simulink model "PVHome"  (R2022b)
settings: Solver=FixedStepDiscrete  StartTime=0.0  StopTime=2  FixedStep=5e-6  RelTol=1e-3
undefined symbols (not defined in the file): Ion, Lithium
libraries: spsSeriesRLCBranchLib x175, spsBreakerLib x103, spsPWMGeneratorDCDCLib x94, spsThyristorLib x78, slpidlib x72, spsIGBTDiodeLib x62, spsThreePhaseVIMeasurementLib x59, spsThreePhaseBreakerLib x45, spsVoltageMeasurementLib x45, spsDiodeLib x39, spsThreePhaseParallelRLCBranchLib x38, spsMosfetLib x32
(part 6 of 16)

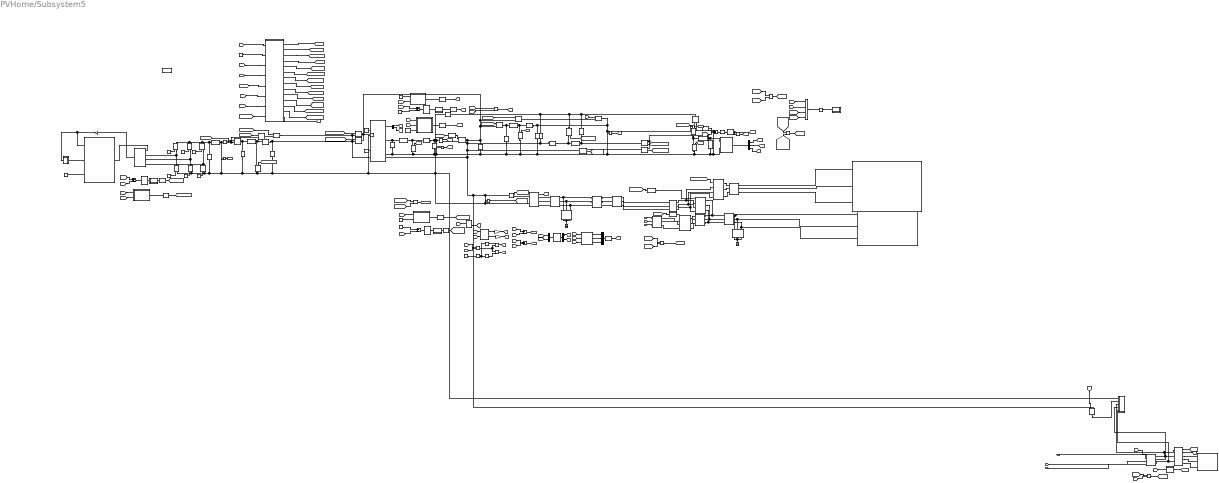
== system PVHome/Subsystem5 ==
  note: CONSUMER
  note: LOAD HOUSE
  note: TRADER GRID
  note: consider a such a language so as to make the system to understand
      |
      | hence consider a system with values range (around keep it as heat) as 0 to 1 but it has to show until 200 degrees.
      |
      | so we divide 1/200 and get 0.005
      |
      | each dividision becomes 0.005
      | 1 is 0.005
      | 2 is 0.01
      | 3 is 0.015
      | 4 is 0.02
      |
      |
      | like that
      | 0.5 becomes 100
      |
      | why not till 200?
      |
      |
      | maybe can increase cost, space like that.
      | hence we program it.
      |
      | consider an integral controller, the default set needed input is around 120 degree and in 0 to 1 scale of 200 divisions (max 200 degree means and 1 is 200).
      |
      | we only get 70 and its 0.35 in set range
      |
      | but we need 120 ie 0.6
      |
      | so the difference becomes error E(t)=50
      | (1/200) integral of E(t) at 0 to t at t=1, it becomes 50(1)/200= 0.25.
      |
      | hence 0.25 must be added to the 0.35 to make it 0.6. so the 0.25 is slowly added to the system with 0.35 and makes it 0.6.
      |
      | after it becomes 0.6, the output is 120 and error is 0 and 0.6 is neither lessened or addened due to past system memory.
      |
      |
      | therefore the 0 to 1 with 200 divisions is a kind of thing that set to make the system understand the human mind from outside.
      |
      | again why not 0 to 200?, human designes the system, consider it has been designed like this.
  note: for how much seconds the output is produced is solver
      | if for 5e-3 seconds in solver a output is loaded for each of 5e-3 seconds
      |
      |
      | powergui is needed because the power system blocks could not be solved using the normal solver.
      |
      | we need a seperate ones like power gui to regulate output within given times.
      |
      | those both normla global solver and the gui must sink such as to make the functions and output possible.
      |
      | or the system cant produce output
      |
      | the gui suppose runs at 4e-3 and normal at 5e-3
      |
      | the output at power system is produced once 4e-3 s
      | and that output is loaded in 5e-3 seconds
      |
      |
      | the synchronzation problem occurs
  note: REAL GRID
  note: Negative meetup
  note: positive total
  note: less act
  note: when th produced voltage supply becomes less than the thought of battery voltage
  note: when the produced voltage becomes high comparitive to the battery
  note: 60
  note: 150
  note: 45
  note: 60
  note: 15
  note: Buck conv
  note: Boost conv
  note: WIND TURBINES
  note: Dc to ac asnd also the Power factor scrutnification
  note: This is for random speeds
  note: Look, the Pu values are nothing but the like example the if at all value is 1, means the value of 3.3 KW is divided into 10 parts. if at all the 0.1 means 10% of 3.3Kw.
      | In turn in the base wind the maximum is 12 and the PU is 1.3, the 13 is divided into 13 parts.
  note: Basically this capacitor works in a way like if at all there is the igbt closed, the capacior will make the higher potential say 190 V and the anode of diode will be 0 V and this makes the capacitor higher potential and anode lower potential and hence reverse bias. After that, when the power flows inside (anode) it, the becomes 230 V suppose, this will surely be higher potential and the 190V will be lower potental and the power flows in forward bias
  note: the tan of the phi and the pi power is Q
  note: Basically in pi controller consider the Default or setted ones are like 120 degree celcius. If at all the feedback input is around 70 degree celcius, the error becomes like 50 degrees. this will go in and the feedback input's magnitude will be considered as the ki as 1/70 and the integral will be from 0 to t as limits and the {E(t)=50}dt inside. Then the 0.42 of error produces and this will make the system increase the 0.42 percet or something. (considering 0.7 before) and goes to 1.142. This will make system at120 degree celcius. This inturn returns as feedback input and the error is 0 and the 1.142 doesnet decrease or increase due to system memory.
  note: basically pitch angle is the one which. Before that, the windmill soins in certain way and in turn the wings of the windmill also rotates. basically like earth rotation is wings and the earth's revolution is the spinning of wings.
      |
      | The pitch angle must be 0 for maximum speed and 90 for minimum speed.
      | the pitch controller is deisgned in such a way that itg included the Pi control mechanism inside it.
      | When the error comes in the PI, kt converts suitable values and proceeeds with into the system via out.
      | After that if at all the output of the system and the refrecnce makes the error 0, thr picth degree stays at specific increases point. or decresaed point.
      |
      |
      |
      | If consider taht the error is  neagtive, then the speed is more than default or setted speed. this makes the RPM to spin fast more than rated speed and making it to damage. Even though the power will wont be produced more , but causes physical damage. Hence that negative causes to increase the pitch angle to certain level (basicallyturn) and make it spin less.
  note: think like a right angled triangle. the hypotenuse as apprarent power, the vertical ones as the VI cos phi that is active power, and the sine ones VI sin phi as the reactive power,
  note: if you remove the cos phi, you will just get the apprarent power which is combination of the active power and reactive power
  note: Trading grid
  note: House Load DC to AC conversion
  note: Battery recharge and discharge system
  note: PV Array System
  note: Centralized system
  note: HOUSE LOAD
  note: so basically these are used like for solving equations. Each type of equation has a each need. the power electronics and other stuff has some other discrete mode and need ans other stuff.
      | the thing at bottom right will evaluate some signal equation only not deep power electronics and stuff.
      | to match those we keep that power gui block. continious signals will help in bothcases and will evaluate.
      | the time is which 5e-6 like how much time interval thse will work
      | the each equation is getting evaluated in this much small interval.
      | the pwm signal around goes upto 50000 cycles in real human second according to this solver
  note: this and the power gui matches then the power system specialized will be resolvered in this sepcific timem like 5e-6
  note: the solver time like 5e-6 will solve each and next equations in this specific time
  note: Like without the power gui the simulink cant simulate the power specializized systems
  note: so these power gui blocks and the solvers are used in such a away that the functions are done
  note: because power (current flows from higher potential to lower potentail
  note: here in capacitor, when the other part of diode is higher potential and this capacior has lower potential, the power flows, if its vice versa, the capacitor side becomes the higher potential and the other side becomes lower potential
  note: breaker analogy
  note: 1 open
  note: 0 closed
  note: Q=VItan phi
  note: phi is cos inverse
  note: Power factor = cos phi
  note: this must activate when there is pv power availablity
  note: this must activate when no power is available in the pv or no sufficient power available in PV
  Add : Sum  Inputs=+-
  Add2 : Sum  Inputs=+-
  Add3 : Sum  Inputs=+-
  Battery : spsBatteryLib/Battery  BatType=Lithium-Ion  ShowTempParam=off  ThermalPreset=no  ShowAgeParam=off  NomV=60  NomQ=50  SOC=50  Batt_Tr=1  PresetModel=off  MaxQ=50  MinV=45  FullV=69.8392  Dis_rate=21.7391  R=0.012  Normal_OP=45.2174  expZone="[64.8232      2.45652]"  current=[6.5 13 32.5]  Units=Time  Tci=20  NomT=20  T2=-30  MaxQ2=4.8  FullV2=7.1  Normal_OP2=5.655  expZone2="[6.58           1]"  Rca=0.6  ti=2000  Dp=0  Neq0=0  Tsim=1e6  Ta1=25  Qeol=5.4*0.9  Reol=0.013333*1.2  Char_age=[2.3478, 3]  Dis_age=[2.3478, 10]  N1=1500  N2=10500  N3=1000  N4=1400  Ta2=45  N5=950
  Breaker{1..10,19} (11 alike) : spsBreakerLib/Breaker  InitialState=0  SwitchingTimes="[1/60  5/60]"  External=on  BreakerResistance=0.01  SnubberResistance=1e6  SnubberCapacitance=inf  Measurements=None  MoreParameters=on  NoBreakLoop=off
  Bus Creator : BusCreator  Inputs=3
  Bus Selector : BusSelector  OutputSignals=V_PV,I_PV
  Bus Selector1 : BusSelector  OutputSignals=SOC (%),Current (A),Voltage (V)
  CAPACITOR {1,7,9..10,14} (5 alike) : spsSeriesRLCBranchLib/Series RLC Branch  LConnTagsString=__new0  RConnTagsString=__new0  BranchType=RC  Resistance=1e-4  Inductance=5e-3  SetiL0=off  InitialCurrent=0  Capacitance=2000e-3  Setx0=off  InitialVoltage=0  Measurements=None
  CAPACITOR {2,8,11,13,18} (5 alike) : spsSeriesRLCBranchLib/Series RLC Branch  LConnTagsString=__new0  RConnTagsString=__new0  BranchType=RL  Resistance=1e-4  Inductance=1e-3  SetiL0=off  InitialCurrent=0  Capacitance=100e-6  Setx0=off  InitialVoltage=0  Measurements=None
  CAPACITOR {3..5,12,16..17,19} (7 alike) : spsSeriesRLCBranchLib/Series RLC Branch  LConnTagsString=__new0  RConnTagsString=__new0  BranchType=RC  Resistance=1e-4  Inductance=5e-3  SetiL0=off  InitialCurrent=0  Capacitance=100e-6  Setx0=off  InitialVoltage=0  Measurements=None
  CAPACITOR 6 : spsSeriesRLCBranchLib/Series RLC Branch  LConnTagsString=__new0  RConnTagsString=__new0  BranchType=RL  Resistance=1e-4  Inductance=13e-3  SetiL0=off  InitialCurrent=0  Capacitance=100e-6  Setx0=off  InitialVoltage=0  Measurements=None
  Centralized System : MATLAB Function  TreatAsAtomicUnit=on
  Constant : Constant  Value=1000
  Constant1 : Constant  Value=25
  Constant2 : Constant  Value=0.005
  Constant3 : Constant  Value=60
  Constant4 : Constant  Value=2300
  Constant5 : Constant  Value=25
  Constant6 : Constant  Value=60
  Current Measurement1 : spsCurrentMeasurementLib/Current Measurement  PhasorSimulation=off  OutputType=Complex  PSBequivalent=0
  Current Measurement2 : spsCurrentMeasurementLib/Current Measurement  PhasorSimulation=off  OutputType=Complex  PSBequivalent=0
  Current Measurement3 : spsCurrentMeasurementLib/Current Measurement  PhasorSimulation=off  OutputType=Complex  PSBequivalent=0
  Data Type Conversion : DataTypeConversion  OutDataTypeStr=boolean  SaturateOnIntegerOverflow=off  RndMeth=Floor
  Data Type Conversion1 : DataTypeConversion  OutDataTypeStr=boolean  SaturateOnIntegerOverflow=off  RndMeth=Floor
  Data Type Conversion2 : DataTypeConversion  OutDataTypeStr=boolean  SaturateOnIntegerOverflow=off  RndMeth=Floor
  Demux : Demux  Outputs=2
  Diode{1..4} (4 alike) : spsDiodeLib/Diode  Ron=0.001  Lon=0  Vf=0.8  IC=0  UseSnubber=0  Rs=500  Cs=250e-9  Measurements=off
  Discrete PID Controller : slpidlib/PID Controller  Controller=PI  Form=Parallel  TimeDomain=Discrete-time  UseExternalTs=off  SampleTime=1e-5  IntegratorMethod=Forward Euler  FilterMethod=Forward Euler  ControllerParametersSource=internal  P=0.01  I=1  UseKiTs=off  D=0  N=100  UseFilter=on  TunerSelectOption=Transfer Function Based (PID Tuner App)  InitialConditionSource=internal  InitialConditionForIntegrator=0  InitialConditionForFilter=0  DifferentiatorICPrevScaledInput=0  ExternalReset=none  TrackingMode=off  Kt=1  LimitOutput=on  SatLimitsSource=internal  UpperSaturationLimit=1.1  LowerSaturationLimit=-1.1  LinearizeAsGain=off  AntiWindupMode=none  Kb=1  LimitIntegrator=off  UpperIntegratorSaturationLimit=inf  LowerIntegratorSaturationLimit=-inf  POutMin=[]  POutMax=[]  IOutMin=[]  IOutMax=[]  DOutMin=[]  DOutMax=[]  NOutMin=[]  NOutMax=[]  SumOutMin=[]  SumOutMax=[]  SaturationOutMin=[]  SaturationOutMax=[]  PParamMin=[]  PParamMax=[]  IParamMin=[]  IParamMax=[]  DParamMin=[]  DParamMax=[]  NParamMin=[]  NParamMax=[]  KbParamMin=[]  KbParamMax=[]  KtParamMin=[]  KtParamMax=[]  KbOutMin=[]  KbOutMax=[]  KtOutMin=[]  KtOutMax=[]  IntegratorOutMin=[]  IntegratorOutMax=[]  FilterOutMin=[]  FilterOutMax=[]  SumI1OutMin=[]  SumI1OutMax=[]  SumI2OutMin=[]  SumI2OutMax=[]  SumI3OutMin=[]  SumI3OutMax=[]  SumI4OutMin=[]  SumI4OutMax=[]  SumDOutMin=[]  SumDOutMax=[]  DifferentiatorOutMin=[]  DifferentiatorOutMax=[]  FilterDiffOutCoefMin=[]  FilterDiffOutCoefMax=[]  ReciprocalOutMin=[]  ReciprocalOutMax=[]  SumDenOutMin=[]  SumDenOutMax=[]  SumNumOutMin=[]  SumNumOutMax=[]  DivideOutMin=[]  DivideOutMax=[]  UdiffTsProdOutMin=[]  UdiffTsProdOutMax=[]  NTsProdOutMin=[]  NTsProdOutMax=[]  UintegralTsProdOutMin=[]  UintegralTsProdOutMax=[]  UngainTsProdOutMin=[]  UngainTsProdOutMax=[]  ClampingZeroOutDataTypeStr=Inherit: Inherit via back propagation  ClampingZeroOutMin=[]  ClampingZeroOutMax=[]  FilterDenConstantOutDataTypeStr=Inherit: Inherit via back propagation  FilterDenConstantOutMin=[]  FilterDenConstantOutMax=[]  PCopyOutDataTypeStr=Inherit: Inherit via back propagation  PCopyOutMin=[]  PCopyOutMax=[]  NCopyOutDataTypeStr=Inherit: Inherit via back propagation  NCopyOutMin=[]  NCopyOutMax=[]  IntegratorContinuousStateAttributes=''  IntegratorStateMustResolveToSignalObject=off  IntegratorRTWStateStorageClass=Auto  FilterContinuousStateAttributes=''  FilterStateMustResolveToSignalObject=off  FilterRTWStateStorageClass=Auto  ParallelPVariant=InternalParameters  IdealPVariant=Disabled  IVariant=InternalParameters  DVariant=Disabled  IntegratorVariant=Discrete  SatVariant=Enabled  AWVariant=Passthrough  PCopyVariant=Disabled  TRVariant=Disabled  FdbkBlocksVariant=Forward  IdealPFdbkVariant=Disabled  SatFdbkVariant=Disabled  DerivativeFilterVariant=Disabled  NVariant=Disabled  NCopyVariant=Disabled_SignalSpec  FilterICVariant=Disabled  IntegratorICVariant=InternalICs  ExternalResetVariant=Disabled  TRSumVariant=Passthrough  SumFdbkVariant=Disabled  SumVariant=Sum_PI  TsampFilterVariant=InternalTs  TsampNgainVariant=Passthrough  TsampIntegralVariant=Passthrough  ExternalSaturationOutDataTypeStr=Inherit: Same as second input
      settings: LibrarySourceBlock=simulink/Discrete/Discrete PID Controller
  Discrete PID Controller1 : slpidlib/PID Controller  Controller=PI  Form=Parallel  TimeDomain=Discrete-time  UseExternalTs=off  SampleTime=-1  IntegratorMethod=Forward Euler  FilterMethod=Forward Euler  ControllerParametersSource=internal  P=1  I=1  UseKiTs=off  D=0  N=100  UseFilter=on  TunerSelectOption=Transfer Function Based (PID Tuner App)  InitialConditionSource=internal  InitialConditionForIntegrator=0  InitialConditionForFilter=0  DifferentiatorICPrevScaledInput=0  ExternalReset=none  TrackingMode=off  Kt=1  LimitOutput=off  SatLimitsSource=internal  UpperSaturationLimit=inf  LowerSaturationLimit=-inf  LinearizeAsGain=off  AntiWindupMode=none  Kb=1  LimitIntegrator=off  UpperIntegratorSaturationLimit=inf  LowerIntegratorSaturationLimit=-inf  POutMin=[]  POutMax=[]  IOutMin=[]  IOutMax=[]  DOutMin=[]  DOutMax=[]  NOutMin=[]  NOutMax=[]  SumOutMin=[]  SumOutMax=[]  SaturationOutMin=[]  SaturationOutMax=[]  PParamMin=[]  PParamMax=[]  IParamMin=[]  IParamMax=[]  DParamMin=[]  DParamMax=[]  NParamMin=[]  NParamMax=[]  KbParamMin=[]  KbParamMax=[]  KtParamMin=[]  KtParamMax=[]  KbOutMin=[]  KbOutMax=[]  KtOutMin=[]  KtOutMax=[]  IntegratorOutMin=[]  IntegratorOutMax=[]  FilterOutMin=[]  FilterOutMax=[]  SumI1OutMin=[]  SumI1OutMax=[]  SumI2OutMin=[]  SumI2OutMax=[]  SumI3OutMin=[]  SumI3OutMax=[]  SumI4OutMin=[]  SumI4OutMax=[]  SumDOutMin=[]  SumDOutMax=[]  DifferentiatorOutMin=[]  DifferentiatorOutMax=[]  FilterDiffOutCoefMin=[]  FilterDiffOutCoefMax=[]  ReciprocalOutMin=[]  ReciprocalOutMax=[]  SumDenOutMin=[]  SumDenOutMax=[]  SumNumOutMin=[]  SumNumOutMax=[]  DivideOutMin=[]  DivideOutMax=[]  UdiffTsProdOutMin=[]  UdiffTsProdOutMax=[]  NTsProdOutMin=[]  NTsProdOutMax=[]  UintegralTsProdOutMin=[]  UintegralTsProdOutMax=[]  UngainTsProdOutMin=[]  UngainTsProdOutMax=[]  ClampingZeroOutDataTypeStr=Inherit: Inherit via back propagation  ClampingZeroOutMin=[]  ClampingZeroOutMax=[]  FilterDenConstantOutDataTypeStr=Inherit: Inherit via back propagation  FilterDenConstantOutMin=[]  FilterDenConstantOutMax=[]  PCopyOutDataTypeStr=Inherit: Inherit via back propagation  PCopyOutMin=[]  PCopyOutMax=[]  NCopyOutDataTypeStr=Inherit: Inherit via back propagation  NCopyOutMin=[]  NCopyOutMax=[]  IntegratorContinuousStateAttributes=''  IntegratorStateMustResolveToSignalObject=off  IntegratorRTWStateStorageClass=Auto  FilterContinuousStateAttributes=''  FilterStateMustResolveToSignalObject=off  FilterRTWStateStorageClass=Auto  ParallelPVariant=InternalParameters  IdealPVariant=Disabled  IVariant=InternalParameters  DVariant=Disabled  IntegratorVariant=Discrete  SatVariant=Disabled  AWVariant=Passthrough  PCopyVariant=Disabled  TRVariant=Disabled  FdbkBlocksVariant=Forward  IdealPFdbkVariant=Disabled  SatFdbkVariant=Disabled  DerivativeFilterVariant=Disabled  NVariant=Disabled  NCopyVariant=Disabled_SignalSpec  FilterICVariant=Disabled  IntegratorICVariant=InternalICs  ExternalResetVariant=Disabled  TRSumVariant=Passthrough  SumFdbkVariant=Disabled  SumVariant=Sum_PI  TsampFilterVariant=InternalTs  TsampNgainVariant=Passthrough  TsampIntegralVariant=Passthrough  ExternalSaturationOutDataTypeStr=Inherit: Same as second input
      settings: LibrarySourceBlock=simulink/Discrete/Discrete PID Controller
  Discrete PID Controller3 : slpidlib/PID Controller  Controller=PI  Form=Parallel  TimeDomain=Discrete-time  UseExternalTs=off  SampleTime=1e-5  IntegratorMethod=Forward Euler  FilterMethod=Forward Euler  ControllerParametersSource=internal  P=0  I=0.01667  UseKiTs=off  D=0  N=100  UseFilter=on  TunerSelectOption=Transfer Function Based (PID Tuner App)  InitialConditionSource=internal  InitialConditionForIntegrator=0  InitialConditionForFilter=0  DifferentiatorICPrevScaledInput=0  ExternalReset=none  TrackingMode=off  Kt=1  LimitOutput=on  SatLimitsSource=internal  UpperSaturationLimit=1.1  LowerSaturationLimit=-1.1  LinearizeAsGain=off  AntiWindupMode=none  Kb=1  LimitIntegrator=off  UpperIntegratorSaturationLimit=inf  LowerIntegratorSaturationLimit=-inf  POutMin=[]  POutMax=[]  IOutMin=[]  IOutMax=[]  DOutMin=[]  DOutMax=[]  NOutMin=[]  NOutMax=[]  SumOutMin=[]  SumOutMax=[]  SaturationOutMin=[]  SaturationOutMax=[]  PParamMin=[]  PParamMax=[]  IParamMin=[]  IParamMax=[]  DParamMin=[]  DParamMax=[]  NParamMin=[]  NParamMax=[]  KbParamMin=[]  KbParamMax=[]  KtParamMin=[]  KtParamMax=[]  KbOutMin=[]  KbOutMax=[]  KtOutMin=[]  KtOutMax=[]  IntegratorOutMin=[]  IntegratorOutMax=[]  FilterOutMin=[]  FilterOutMax=[]  SumI1OutMin=[]  SumI1OutMax=[]  SumI2OutMin=[]  SumI2OutMax=[]  SumI3OutMin=[]  SumI3OutMax=[]  SumI4OutMin=[]  SumI4OutMax=[]  SumDOutMin=[]  SumDOutMax=[]  DifferentiatorOutMin=[]  DifferentiatorOutMax=[]  FilterDiffOutCoefMin=[]  FilterDiffOutCoefMax=[]  ReciprocalOutMin=[]  ReciprocalOutMax=[]  SumDenOutMin=[]  SumDenOutMax=[]  SumNumOutMin=[]  SumNumOutMax=[]  DivideOutMin=[]  DivideOutMax=[]  UdiffTsProdOutMin=[]  UdiffTsProdOutMax=[]  NTsProdOutMin=[]  NTsProdOutMax=[]  UintegralTsProdOutMin=[]  UintegralTsProdOutMax=[]  UngainTsProdOutMin=[]  UngainTsProdOutMax=[]  ClampingZeroOutDataTypeStr=Inherit: Inherit via back propagation  ClampingZeroOutMin=[]  ClampingZeroOutMax=[]  FilterDenConstantOutDataTypeStr=Inherit: Inherit via back propagation  FilterDenConstantOutMin=[]  FilterDenConstantOutMax=[]  PCopyOutDataTypeStr=Inherit: Inherit via back propagation  PCopyOutMin=[]  PCopyOutMax=[]  NCopyOutDataTypeStr=Inherit: Inherit via back propagation  NCopyOutMin=[]  NCopyOutMax=[]  IntegratorContinuousStateAttributes=''  IntegratorStateMustResolveToSignalObject=off  IntegratorRTWStateStorageClass=Auto  FilterContinuousStateAttributes=''  FilterStateMustResolveToSignalObject=off  FilterRTWStateStorageClass=Auto  ParallelPVariant=InternalParameters  IdealPVariant=Disabled  IVariant=InternalParameters  DVariant=Disabled  IntegratorVariant=Discrete  SatVariant=Enabled  AWVariant=Passthrough  PCopyVariant=Disabled  TRVariant=Disabled  FdbkBlocksVariant=Forward  IdealPFdbkVariant=Disabled  SatFdbkVariant=Disabled  DerivativeFilterVariant=Disabled  NVariant=Disabled  NCopyVariant=Disabled_SignalSpec  FilterICVariant=Disabled  IntegratorICVariant=InternalICs  ExternalResetVariant=Disabled  TRSumVariant=Passthrough  SumFdbkVariant=Disabled  SumVariant=Sum_PI  TsampFilterVariant=InternalTs  TsampNgainVariant=Passthrough  TsampIntegralVariant=Passthrough  ExternalSaturationOutDataTypeStr=Inherit: Same as second input
      settings: LibrarySourceBlock=simulink/Discrete/Discrete PID Controller
  Discrete PID Controller4 : slpidlib/PID Controller  Controller=PI  Form=Parallel  TimeDomain=Discrete-time  UseExternalTs=off  SampleTime=1e-5  IntegratorMethod=Forward Euler  FilterMethod=Forward Euler  ControllerParametersSource=internal  P=0  I=0.01  UseKiTs=off  D=0  N=100  UseFilter=on  TunerSelectOption=Transfer Function Based (PID Tuner App)  InitialConditionSource=internal  InitialConditionForIntegrator=0  InitialConditionForFilter=0  DifferentiatorICPrevScaledInput=0  ExternalReset=none  TrackingMode=off  Kt=1  LimitOutput=on  SatLimitsSource=internal  UpperSaturationLimit=1.1  LowerSaturationLimit=-1.1  LinearizeAsGain=off  AntiWindupMode=none  Kb=1  LimitIntegrator=off  UpperIntegratorSaturationLimit=inf  LowerIntegratorSaturationLimit=-inf  POutMin=[]  POutMax=[]  IOutMin=[]  IOutMax=[]  DOutMin=[]  DOutMax=[]  NOutMin=[]  NOutMax=[]  SumOutMin=[]  SumOutMax=[]  SaturationOutMin=[]  SaturationOutMax=[]  PParamMin=[]  PParamMax=[]  IParamMin=[]  IParamMax=[]  DParamMin=[]  DParamMax=[]  NParamMin=[]  NParamMax=[]  KbParamMin=[]  KbParamMax=[]  KtParamMin=[]  KtParamMax=[]  KbOutMin=[]  KbOutMax=[]  KtOutMin=[]  KtOutMax=[]  IntegratorOutMin=[]  IntegratorOutMax=[]  FilterOutMin=[]  FilterOutMax=[]  SumI1OutMin=[]  SumI1OutMax=[]  SumI2OutMin=[]  SumI2OutMax=[]  SumI3OutMin=[]  SumI3OutMax=[]  SumI4OutMin=[]  SumI4OutMax=[]  SumDOutMin=[]  SumDOutMax=[]  DifferentiatorOutMin=[]  DifferentiatorOutMax=[]  FilterDiffOutCoefMin=[]  FilterDiffOutCoefMax=[]  ReciprocalOutMin=[]  ReciprocalOutMax=[]  SumDenOutMin=[]  SumDenOutMax=[]  SumNumOutMin=[]  SumNumOutMax=[]  DivideOutMin=[]  DivideOutMax=[]  UdiffTsProdOutMin=[]  UdiffTsProdOutMax=[]  NTsProdOutMin=[]  NTsProdOutMax=[]  UintegralTsProdOutMin=[]  UintegralTsProdOutMax=[]  UngainTsProdOutMin=[]  UngainTsProdOutMax=[]  ClampingZeroOutDataTypeStr=Inherit: Inherit via back propagation  ClampingZeroOutMin=[]  ClampingZeroOutMax=[]  FilterDenConstantOutDataTypeStr=Inherit: Inherit via back propagation  FilterDenConstantOutMin=[]  FilterDenConstantOutMax=[]  PCopyOutDataTypeStr=Inherit: Inherit via back propagation  PCopyOutMin=[]  PCopyOutMax=[]  NCopyOutDataTypeStr=Inherit: Inherit via back propagation  NCopyOutMin=[]  NCopyOutMax=[]  IntegratorContinuousStateAttributes=''  IntegratorStateMustResolveToSignalObject=off  IntegratorRTWStateStorageClass=Auto  FilterContinuousStateAttributes=''  FilterStateMustResolveToSignalObject=off  FilterRTWStateStorageClass=Auto  ParallelPVariant=InternalParameters  IdealPVariant=Disabled  IVariant=InternalParameters  DVariant=Disabled  IntegratorVariant=Discrete  SatVariant=Enabled  AWVariant=Passthrough  PCopyVariant=Disabled  TRVariant=Disabled  FdbkBlocksVariant=Forward  IdealPFdbkVariant=Disabled  SatFdbkVariant=Disabled  DerivativeFilterVariant=Disabled  NVariant=Disabled  NCopyVariant=Disabled_SignalSpec  FilterICVariant=Disabled  IntegratorICVariant=InternalICs  ExternalResetVariant=Disabled  TRSumVariant=Passthrough  SumFdbkVariant=Disabled  SumVariant=Sum_PI  TsampFilterVariant=InternalTs  TsampNgainVariant=Passthrough  TsampIntegralVariant=Passthrough  ExternalSaturationOutDataTypeStr=Inherit: Same as second input
      settings: LibrarySourceBlock=simulink/Discrete/Discrete PID Controller
  Discrete PID Controller5 : slpidlib/PID Controller  Controller=PI  Form=Parallel  TimeDomain=Discrete-time  UseExternalTs=off  SampleTime=1e-5  IntegratorMethod=Forward Euler  FilterMethod=Forward Euler  ControllerParametersSource=internal  P=0  I=0.01  UseKiTs=off  D=0  N=100  UseFilter=on  TunerSelectOption=Transfer Function Based (PID Tuner App)  InitialConditionSource=internal  InitialConditionForIntegrator=0  InitialConditionForFilter=0  DifferentiatorICPrevScaledInput=0  ExternalReset=none  TrackingMode=off  Kt=1  LimitOutput=on  SatLimitsSource=internal  UpperSaturationLimit=1.1  LowerSaturationLimit=-1.1  LinearizeAsGain=off  AntiWindupMode=none  Kb=1  LimitIntegrator=off  UpperIntegratorSaturationLimit=inf  LowerIntegratorSaturationLimit=-inf  POutMin=[]  POutMax=[]  IOutMin=[]  IOutMax=[]  DOutMin=[]  DOutMax=[]  NOutMin=[]  NOutMax=[]  SumOutMin=[]  SumOutMax=[]  SaturationOutMin=[]  SaturationOutMax=[]  PParamMin=[]  PParamMax=[]  IParamMin=[]  IParamMax=[]  DParamMin=[]  DParamMax=[]  NParamMin=[]  NParamMax=[]  KbParamMin=[]  KbParamMax=[]  KtParamMin=[]  KtParamMax=[]  KbOutMin=[]  KbOutMax=[]  KtOutMin=[]  KtOutMax=[]  IntegratorOutMin=[]  IntegratorOutMax=[]  FilterOutMin=[]  FilterOutMax=[]  SumI1OutMin=[]  SumI1OutMax=[]  SumI2OutMin=[]  SumI2OutMax=[]  SumI3OutMin=[]  SumI3OutMax=[]  SumI4OutMin=[]  SumI4OutMax=[]  SumDOutMin=[]  SumDOutMax=[]  DifferentiatorOutMin=[]  DifferentiatorOutMax=[]  FilterDiffOutCoefMin=[]  FilterDiffOutCoefMax=[]  ReciprocalOutMin=[]  ReciprocalOutMax=[]  SumDenOutMin=[]  SumDenOutMax=[]  SumNumOutMin=[]  SumNumOutMax=[]  DivideOutMin=[]  DivideOutMax=[]  UdiffTsProdOutMin=[]  UdiffTsProdOutMax=[]  NTsProdOutMin=[]  NTsProdOutMax=[]  UintegralTsProdOutMin=[]  UintegralTsProdOutMax=[]  UngainTsProdOutMin=[]  UngainTsProdOutMax=[]  ClampingZeroOutDataTypeStr=Inherit: Inherit via back propagation  ClampingZeroOutMin=[]  ClampingZeroOutMax=[]  FilterDenConstantOutDataTypeStr=Inherit: Inherit via back propagation  FilterDenConstantOutMin=[]  FilterDenConstantOutMax=[]  PCopyOutDataTypeStr=Inherit: Inherit via back propagation  PCopyOutMin=[]  PCopyOutMax=[]  NCopyOutDataTypeStr=Inherit: Inherit via back propagation  NCopyOutMin=[]  NCopyOutMax=[]  IntegratorContinuousStateAttributes=''  IntegratorStateMustResolveToSignalObject=off  IntegratorRTWStateStorageClass=Auto  FilterContinuousStateAttributes=''  FilterStateMustResolveToSignalObject=off  FilterRTWStateStorageClass=Auto  ParallelPVariant=InternalParameters  IdealPVariant=Disabled  IVariant=InternalParameters  DVariant=Disabled  IntegratorVariant=Discrete  SatVariant=Enabled  AWVariant=Passthrough  PCopyVariant=Disabled  TRVariant=Disabled  FdbkBlocksVariant=Forward  IdealPFdbkVariant=Disabled  SatFdbkVariant=Disabled  DerivativeFilterVariant=Disabled  NVariant=Disabled  NCopyVariant=Disabled_SignalSpec  FilterICVariant=Disabled  IntegratorICVariant=InternalICs  ExternalResetVariant=Disabled  TRSumVariant=Passthrough  SumFdbkVariant=Disabled  SumVariant=Sum_PI  TsampFilterVariant=InternalTs  TsampNgainVariant=Passthrough  TsampIntegralVariant=Passthrough  ExternalSaturationOutDataTypeStr=Inherit: Same as second input
      settings: LibrarySourceBlock=simulink/Discrete/Discrete PID Controller
  Divide{,1..8} (9 alike) : Product  Inputs=**
  Gain : Gain
  Ground : spsGroundLib/Ground  LConnTagsString=a
  Ground1 : spsGroundLib/Ground  LConnTagsString=a
  IGBT/Diode{,1..5} (6 alike) : spsIGBTDiodeLib/IGBT//Diode  Ron=1e-3  Rs=1e5  Cs=inf  Measurements=off
  MATLAB Function : MATLAB Function  TreatAsAtomicUnit=on
  MATLAB Function1 : MATLAB Function  TreatAsAtomicUnit=on
  MATLAB Function2 : MATLAB Function  TreatAsAtomicUnit=on
  MATLAB Function3 : MATLAB Function  TreatAsAtomicUnit=on
  MATLAB Function4 : MATLAB Function  TreatAsAtomicUnit=on
  MATLAB Function5 : MATLAB Function  TreatAsAtomicUnit=on
  MATLAB Function6 : MATLAB Function  TreatAsAtomicUnit=on
  MATLAB Function7 : MATLAB Function  TreatAsAtomicUnit=on
  MATLAB Function8 : MATLAB Function  TreatAsAtomicUnit=on
  MATLAB Function9 : MATLAB Function  TreatAsAtomicUnit=on
  Mosfet : spsMosfetLib/Mosfet  Ron=0.1  Lon=0  Rd=0.01  Vfd=0  IC=0  Rs=1e5  Cs=inf  Measurements=off
  Mosfet1 : spsMosfetLib/Mosfet  Ron=0.1  Lon=0  Rd=0.01  Vfd=0  IC=0  Rs=1e5  Cs=inf  Measurements=off
  Mosfet2 : spsMosfetLib/Mosfet  Ron=0.1  Lon=0  Rd=0.01  Vfd=0  IC=0  Rs=1e5  Cs=inf  Measurements=off
  Mux : Mux  Inputs=2
  Mux1 : Mux
  NOT : Logic  Operator=NOT  IconShape=distinctive  AllPortsSameDT=off  OutDataTypeStr=boolean
  PF : Constant  Value=0.99
  PLL (3ph) : spsPLL3phLib/PLL (3ph)  Fmin=60  Par_Init=[0, 50]  ParK=[180, 3200, 1]  TcD=1e-4  MaxRateChangeFreq=12  FilterCutOffFreq=25  Ts=1e-5  AGC=on
  PV Array : spsPVArrayLib/PV Array  Npar=4  Nser=4  PlotType=array @ 1000 W/m2 & specified temperatures  S_vec="[ 1000  500  100 ]"  Temp_C_vec="[ 45 25  ]"  ModuleName=User-defined  PlotWhenSelected=off  Pm=213.15  Ncell=60  Voc=36.3  Isc=7.84  Vm=29  Im=7.35  beta_Voc_pc=-0.36099  alpha_Isc_pc=0.102  beta_Voc=-0.13104  alpha_Isc=0.0079968  IL=7.8654  I0=2.9273e-10  nI=0.98119  Rsh=313.0553  Rs=0.39381  RobustModel=off  RobustCellTemperature=313.3991  BAL=on  Tc=1e-6  Tfilter=5e-5
  PWM Generator (2-Level) : spsPWMGenerator2LevelLib/PWM Generator (2-Level)  ModulatorType=Three-phase bridge (6 pulses)  ModulatorMode=Unsynchronized  Fc=27*60  Pc=90  nF=27  MinMax="[ -1  1 ]"  SamplingTechnique=Natural  ModulatingSignals=off  m=0.8  Freq=60  Phase=0  Ts=1e-5  ShowCarrierOutport=off
  PWM Generator (DC-DC) : spsPWMGeneratorDCDCLib/PWM Generator (DC-DC)  Fsw=20000  Ts=5e-6
  PWM Generator (DC-DC){1..6,8} (7 alike) : spsPWMGeneratorDCDCLib/PWM Generator (DC-DC)  Fsw=10000  Ts=5e-6
  Permanent Magnet Synchronous Machine : spsPermanentMagnetSynchronousMachineLib/Permanent Magnet Synchronous Machine  NbPhases=3  FluxDistribution=Sinusoidal  RotorType=Round  MechanicalLoad=Torque Tm  PresetModel=No  ShowDetailedParameters=on  MeasurementBus=off  Resistance=0.0485  Inductance=8.5e-3  dqInductances=[8.5e-3,8.5e-3]  La=0.000395  MachineConstant=Flux linkage established by magnets (V.s)  Flux=0.1194  VoltageCst=86.6271  TorqueCst=0.7164  Flat=120  Mechanical=[0.0027 0.0004924 4 0]  PolePairs=4  InitialConditions=[0,0, 0,0]  InitialConditions5ph=[0 0 0 0 0 0]  RefAngle=90 degrees behind phase A axis (modified Park)  IterativeDiscreteModel=Trapezoidal non iterative  TsBlock=-1  TsPowergui=0
  Pitch Controller : Subsystem
  "Power (3ph, Instantaneous)" : spsPower3phInstantaneousLib/Power (3ph, Instantaneous)
  Pulse Generator : DiscretePulseGenerator  PulseType=Time based  Period=0.02  PulseWidth=10  PhaseDelay=0*0.02/360
  Pulse Generator1 : DiscretePulseGenerator  PulseType=Time based  Period=0.02  PulseWidth=10  PhaseDelay=(0+60)*0.02/360
  Pulse Generator2 : DiscretePulseGenerator  PulseType=Time based  Period=0.02  PulseWidth=10  PhaseDelay=(0+120)*0.02/360
  Pulse Generator3 : DiscretePulseGenerator  PulseType=Time based  Period=0.02  PulseWidth=10  PhaseDelay=(0+180)*0.02/360
  Pulse Generator4 : DiscretePulseGenerator  PulseType=Time based  Period=0.02  PulseWidth=10  PhaseDelay=(0+240)*0.02/360
  Pulse Generator5 : DiscretePulseGenerator  PulseType=Time based  Period=0.02  PulseWidth=10  PhaseDelay=(0+360)*0.02/360
  Repeating Sequence : simulink/Sources/Repeating Sequence  rep_seq_t=[0 1 2 3 4]  rep_seq_y=[0 1 2 3 4]
  Subsystem : Subsystem
  Subtract : Sum  Inputs=+-
  Subtract1 : Sum  Inputs=+-
  Subtract2 : Sum  Inputs=+-
  Supply1 : Constant  Value=60
  Supply2 : Constant  Value=60
  Three phase Inductor removes ripples : spsThreePhaseParallelRLCBranchLib/Three-Phase Parallel RLC Branch  LConnTagsString=A|B|C  RConnTagsString=A|B|C  BranchType=RL  Resistance=0.01  Inductance=1e-6  Capacitance=1e-6  Measurements=None
  Three phase Inductor removes ripples1 : spsThreePhaseParallelRLCBranchLib/Three-Phase Parallel RLC Branch  LConnTagsString=A|B|C  RConnTagsString=A|B|C  BranchType=RC  Resistance=0.01  Inductance=1e-6  Capacitance=1e-6  Measurements=None
  Three phase Inductor removes ripples2 : spsThreePhaseParallelRLCBranchLib/Three-Phase Parallel RLC Branch  LConnTagsString=A|B|C  RConnTagsString=A|B|C  BranchType=RL  Resistance=0.01  Inductance=1e-6  Capacitance=1e-6  Measurements=None
  Three phase Inductor removes ripples3 : spsThreePhaseParallelRLCBranchLib/Three-Phase Parallel RLC Branch  LConnTagsString=A|B|C  RConnTagsString=A|B|C  BranchType=RC  Resistance=0.01  Inductance=1e-6  Capacitance=1e-6  Measurements=None
  Three-Phase Series RLC Load : spsThreePhaseSeriesRLCLoadLib/Three-Phase Series RLC Load  LConnTagsString=A|B|C  Configuration=Y (grounded)  NominalVoltage=400  Vabc=[1e3 1e3 1e3]  Vabcp=[1e3 1e3 1e3]  NominalFrequency=60  UnbalancedPower=off  ActivePower=2300  InductivePower=1.5  CapacitivePower=0  Pabc=[10e3 9e3 11e3]  QLabc=[100 90 110]  QCabc=[100 90 110]  Pabcp=[10e3 9e3 11e3]  QLabcp=[100 90 110]  QCabcp=[100 90 110]  Measurements=Branch voltages and currents  LoadType=constant Z
  Three-Phase V-I Measurement : spsThreePhaseVIMeasurementLib/Three-Phase V-I Measurement  VoltageMeasurement=phase-to-ground  SetLabelV=on  LabelV=VH1_3  Vpu=off  VpuLL=off  CurrentMeasurement=yes  SetLabelI=on  LabelI=IH1_3  Ipu=off  Pbase=100e6  Vbase=500e3  OutputType=Complex  PhasorSimulation=off  PSBequivalent=0
  Three-Phase V-I Measurement1 : spsThreePhaseVIMeasurementLib/Three-Phase V-I Measurement  VoltageMeasurement=phase-to-ground  SetLabelV=on  LabelV=Vgrid_3  Vpu=off  VpuLL=off  CurrentMeasurement=yes  SetLabelI=on  LabelI=Igrid_3  Ipu=off  Pbase=100e6  Vbase=500e3  OutputType=Complex  PhasorSimulation=off  PSBequivalent=0
  Three-Phase V-I Measurement2 : spsThreePhaseVIMeasurementLib/Three-Phase V-I Measurement  VoltageMeasurement=phase-to-ground  SetLabelV=on  LabelV=V_Real_Grid  Vpu=off  VpuLL=off  CurrentMeasurement=yes  SetLabelI=on  LabelI=I_Real_Grid  Ipu=off  Pbase=100e6  Vbase=500e3  OutputType=Complex  PhasorSimulation=off  PSBequivalent=0
  Three-Phase V-I Measurement3 : spsThreePhaseVIMeasurementLib/Three-Phase V-I Measurement  VoltageMeasurement=phase-to-ground  SetLabelV=on  LabelV=V_Grid_Energy_Trade  Vpu=off  VpuLL=off  CurrentMeasurement=yes  SetLabelI=on  LabelI=I_Grid_Energy_Trade  Ipu=off  Pbase=100e6  Vbase=500e3  OutputType=Complex  PhasorSimulation=off  PSBequivalent=0
  Three-Phase V-I Measurement4 : spsThreePhaseVIMeasurementLib/Three-Phase V-I Measurement  VoltageMeasurement=phase-to-ground  SetLabelV=on  LabelV=V_Real_Grid_Grid  Vpu=off  VpuLL=off  CurrentMeasurement=yes  SetLabelI=on  LabelI=I_Real_Grid_Grid  Ipu=off  Pbase=100e6  Vbase=500e3  OutputType=Complex  PhasorSimulation=off  PSBequivalent=0
  Three-Phase V-I Measurement5 : spsThreePhaseVIMeasurementLib/Three-Phase V-I Measurement  VoltageMeasurement=phase-to-ground  SetLabelV=off  LabelV=Vabc  Vpu=off  VpuLL=off  CurrentMeasurement=yes  SetLabelI=off  LabelI=Iabc  Ipu=off  Pbase=100e6  Vbase=500e3  OutputType=Complex  PhasorSimulation=off  PSBequivalent=0
  Three-Phase Breaker : spsThreePhaseBreakerLib/Three-Phase Breaker  InitialState=closed  SwitchA=on  SwitchB=on  SwitchC=on  SwitchTimes="[1/50  10]"  External=off  BreakerResistance=0.01  SnubberResistance=1e6  SnubberCapacitance=inf  Measurements=None
  Three-Phase Breaker{1..4} (4 alike) : spsThreePhaseBreakerLib/Three-Phase Breaker  InitialState=open  SwitchA=on  SwitchB=on  SwitchC=on  SwitchTimes="[1/50  10]"  External=on  BreakerResistance=0.01  SnubberResistance=1e6  SnubberCapacitance=inf  Measurements=None
  Three-Phase Fault : spsThreePhaseFaultLib/Three-Phase Fault  InitialStates=0  FaultA=on  FaultB=on  FaultC=on  GroundFault=on  SwitchTimes=[5 5.1]  External=off  SwitchStatus=NaN  FaultResistance=0.001  GroundResistance=0.01  SnubberResistance=1e6  SnubberCapacitance=inf  Measurements=None
  Three-Phase Source1 : spsThreePhaseSourceLib/Three-Phase Source  InternalConnection=Yg  VoltagePhases=off  Voltage=400  PhaseAngle=0  Voltage_phases=[25e3 25e3 25e3]/sqrt(3)  PhaseAngles_phases=[0 -120 +120]  Frequency=60  NonIdealSource=on  SpecifyImpedance=off  Resistance=0.8929  Inductance=16.58e-3  ShortCircuitLevel=100e6  BaseVoltage=25e3  XRratio=7  BusType=swing  Pref=10e3  Qref=0  Prefabc=[10e3, 10e3, 10e3]  Qrefabc=[0, 0, 0]  Qmin=-inf  Qmax=inf
  Thyristor{,1..5} (6 alike) : spsThyristorLib/Thyristor  Ron=0.001  Lon=0  Vf=0.8  IC=0  Rs=500  Cs=250e-9  Measurements=off
  Trigonometric Function : Trigonometry  Operator=acos
  Trigonometric Function1 : Trigonometry
  Trigonometric Function2 : Trigonometry  Operator=cos
  Universal Bridge : spsUniversalBridgeLib/Universal Bridge  Arms=3  SnubberResistance=1e5  SnubberCapacitance=inf  Device=Thyristors  Ron=1e-3  Lon=0  ForwardVoltages="[  0  0  ]"  ForwardVoltage=0  GTOparameters=[ 10e-6 , 20e-6 ]  IGBTparameters=[ 1e-6 , 2e-6 ]  Measurements=None  Measurements_2=None  converterType=Rectifier
  Voltage Measurement{,1..4} (5 alike) : spsVoltageMeasurementLib/Voltage Measurement  PhasorSimulation=off  OutputType=Complex  PSBequivalent=0
  Wind Turbine : spsWindTurbineLib/Wind Turbine  Pnom=3e3  Pelec_base=3e3/0.9  wind_base=12  P_wind_base=1  speed_nom=1.3  pitch_angle=0  c1_c6="[0.51763          116          0.4            5           21     0.006795]"  cp_nom=0.48  lambda_nom=8.1
  Zero-Order Hold : ZeroOrderHold  SampleTime=0.3
  kVAR : Gain  Gain=1/1000
  kW : Gain  Gain=1/1000
  powergui1 : spspowerguiLib/powergui  Priority=1  SimulationMode=Discrete  SampleTime=5e-6  frequency=60  Iterations=50  frequencyindice=60  Pbase=100e6  ErrMax=1e-4  UnitsV=kV  UnitsW=MW  buscounter=0  FunctionMessages=off  echomessages=off  EnableUseOfTLC=off  CurrentSourceSwitches=off  DisableSnubberDevices=off  DisableRonSwitches=off  DisableVfSwitches=off  DisplayEquations=off  AutomaticDiscreteSolvers=off  SolverType=Tustin/Backward Euler (TBE)  Interpol=off  ExternalGateDelay=off  methode=off  Ts=100  x0status=blocks  SPID=on  SwTol=0  HookPort=off  NonlinearTolerance=1e-4  nMaxIteration=100  ContinueOnMaxIteration=off  RestoreLinks=warning  ResistiveCurrentMeasurement=off  Frange=[0:2:500]  Ylog=off  Xlog=on  ShowGrid=off  save=off  variable=ZData  structure=0  ZoomFFT=off  StartTime=0.0  cycles=1  DisplayStyle=1  fundamental=60  FreqAxis=off  MaxFrequency=1000  frequencyindicesteady=1  RmsSteady=1  display=off
  A : PMIOPort  Side=Left
  B : PMIOPort  Port=2  Side=Left
  C : PMIOPort  Port=3  Side=Left
  A1 : PMIOPort  Port=4  Side=Left
  B1 : PMIOPort  Port=5  Side=Left
  C1 : PMIOPort  Port=6  Side=Left
  wires:
  [Q_ref] -> Subtract1/1
  Demux/1 -> [ma]
  [Vgrid_3] -> PLL (3ph)/1
  [H1_Grid_Circuit_Breaker] -> Data Type Conversion/1
  [PV_H_1] -> IGBT/Diode/1
  [IH1_3] -> "Power (3ph, Instantaneous)"/2
  [PWM_H1] -> Universal Bridge/1
  "Power (3ph, Instantaneous)"/2 -> kVAR/1
  [Ipv] -> MATLAB Function/2(I_PV)
  Bus Selector/1 -> [Vpv]  "<V_PV>"
  [I_PV_1] -> Divide/1
  MATLAB Function/1(duty) -> PWM Generator (DC-DC)/1
  Battery/1 -> Bus Selector1/1
  Trigonometric Function1/1 -> Divide1/2
  [H1_B_Ground_Discharge] -> Breaker3/1
  [P] -> Subtract/2
  Divide5/1 -> Divide1/1, Divide6/2
  PV Array/1 -> Bus Selector/1
  Divide/1 -> [P_Pv]
  Voltage Measurement1/1 -> [V_PV_1]
  Constant/1 -> PV Array/1
  [V_PV_1] -> Divide/2
  Bus Creator/1 -> PWM Generator (2-Level)/1
  [Q_Error] -> Mux/2
  "Power (3ph, Instantaneous)"/1 -> kW/1
  Discrete PID Controller/1 -> Demux/1
  kVAR/1 -> [Q]
  Discrete PID Controller1/1 -> PWM Generator (DC-DC)2/1
  [H1_Grid_Breaker] -> Data Type Conversion1/1
  Bus Selector1/2 -> [IbH1]  "<Current (A)>"
  Bus Selector1/3 -> [VbH1]  "<Voltage (V)>"
  PWM Generator (DC-DC)1/1 -> [BH1]
  [P_ref] -> Subtract/1
  PLL (3ph)/2 -> [wt]
  Subtract/1 -> [P_Error]
  Bus Selector/2 -> [Ipv]  "<I_PV>"
  Current Measurement2/1 -> [I_PV_1]
  PF/1 -> Trigonometric Function/1
  Subtract1/1 -> [Q_Error]
  PWM Generator (DC-DC)/1 -> [PV_H_1]
  [P_Error] -> Mux/1
  Mux/1 -> Discrete PID Controller/1
  [Q] -> Subtract1/2
  [shift] -> MATLAB Function2/3(shift_k)
  Data Type Conversion1/1 -> ?
  PWM Generator (2-Level)/1 -> [PWM_H1]
  MATLAB Function2/3(c) -> Bus Creator/3
  kW/1 -> [P]
  MATLAB Function2/2(b) -> Bus Creator/2
  MATLAB Function2/1(a) -> Bus Creator/1
  [Vpv] -> MATLAB Function/1(V_PV)
  [wt] -> MATLAB Function2/1(x)
  [H1_Pv_Breaker] -> Data Type Conversion2/1
  Data Type Conversion2/1 -> Breaker1/1
  Divide1/1 -> [Q_ref]
  PWM Generator (DC-DC)2/1 -> [P_H1_B], NOT/1
  Data Type Conversion/1 -> ?
  Demux/2 -> [shift]
  Trigonometric Function/1 -> Trigonometric Function1/1, Trigonometric Function2/1
  [VH1_3] -> "Power (3ph, Instantaneous)"/1
  Constant1/1 -> PV Array/2
  [IbH1] -> Add/2
  Constant5/1 -> Add/1
  [N_H1_B] -> IGBT/Diode2/1
  Constant2/1 -> MATLAB Function/3(deltaD)
  NOT/1 -> [N_H1_B]
  [P_H1_B] -> IGBT/Diode1/1
  [ma] -> MATLAB Function2/2(ma)
  Bus Selector1/1 -> [SOCbH1]  "<SOC (%)>"
  [Bi_B_Breaker_Discharge_Boost] -> Breaker4/1
  Add/1 -> Discrete PID Controller1/1
  [V_PV_1] -> MATLAB Function9/1(V_PV_1)
  Supply1/1 -> MATLAB Function9/2(Sixty)
  MATLAB Function9/1(Wind_Breaker_Boost_Signal_Out) -> PWM Generator (DC-DC)3/1
  PWM Generator (DC-DC)3/1 -> [battery_boost_pwm]
  [battery_buck_pwm] -> Mosfet1/1
  Supply2/1 -> Add2/1
  [V_PV_1] -> Add2/2
  Add2/1 -> Discrete PID Controller3/1
  [Bi_B_Breaker_Discharge_Buck] -> Breaker5/1
  [battery_boost_pwm] -> IGBT/Diode4/1
  [V_PV_1] -> Add3/1
  Constant6/1 -> Add3/2
  [SOCbH1] -> Mux1/1
  [P_Pv] -> Mux1/2
  [V_Real_Grid] -> Divide3/1
  [I_Real_Grid] -> Divide3/2
  Divide3/1 -> [Grid_Real_Power]  "Grid_"
  [Grid_Real_Power] -> Mux1/3
  [V_Grid_Energy_Trade] -> Divide4/1
  [I_Grid_Energy_Trade] -> Divide4/2
  Divide4/1 -> [Grid_Trade_Power]  "Grid_"
  [Grid_Trade_Power] -> Mux1/4
  Mux1/1 -> Zero-Order Hold/1
  Zero-Order Hold/1 -> MATLAB Function1/1(u)
  Add3/1 -> Discrete PID Controller4/1
  Discrete PID Controller4/1 -> MATLAB Function3/1(u)
  MATLAB Function3/1(y) -> PWM Generator (DC-DC)1/1
  [BH1] -> Mosfet/1
  Voltage Measurement/1 -> [V1]
  Trigonometric Function2/1 -> Divide6/1
  Divide6/1 -> [P_ref]
  Repeating Sequence/1 -> Wind Turbine/3
  Pitch Controller/1(Out1) -> Wind Turbine/2
  Gain/1 -> Wind Turbine/1, Pitch Controller/1(In1)
  Wind Turbine/1 -> Permanent Magnet Synchronous Machine/1
  Pulse Generator3/1 -> Thyristor3/1
  Pulse Generator2/1 -> Thyristor5/1
  Pulse Generator4/1 -> Thyristor4/1
  Pulse Generator5/1 -> Thyristor2/1
  Pulse Generator1/1 -> Thyristor1/1
  Voltage Measurement3/1 -> [V_Wind]
  Current Measurement1/1 -> [I_Wind]
  Current Measurement3/1 -> [Full_Ren_Current]
  Voltage Measurement4/1 -> [Full_Ren_Voltage]
  [Full_Ren_Current] -> Divide8/1
  [Full_Ren_Voltage] -> Divide8/2
  Divide8/1 -> [Full_Ren_Power]
  [V_Wind] -> Subtract2/1
  [V_PV_1] -> Subtract2/2
  Subtract2/1 -> Discrete PID Controller5/1
  PWM Generator (DC-DC)5/1 -> [Wind_Breaker_Buck_Siganl]
  PWM Generator (DC-DC)6/1 -> [Wind_Breaker_Boost_Signal]
  [Wind_Power_Battery_Breaker_Boost] -> Breaker8/1
  Pulse Generator/1 -> Thyristor/1
  [Wind_Breaker_Boost] -> Breaker6/1
  [Wind_Breaker_Buck] -> Breaker7/1
  [Wind_Breaker_Buck_Siganl] -> Mosfet2/1
  [Wind_Breaker_Boost_Signal] -> IGBT/Diode3/1
  [Wind_Power_Battery_Breaker_Buck] -> Breaker9/1
  [Bi_B_Charge_Breaker_Buck] -> Breaker2/1
  [Bi_B_Charge_Breaker_Boost] -> Breaker10/1
  [BH2] -> IGBT/Diode5/1
  Voltage Measurement2/1 -> [Battery_Passing_Voltage]
  [VH1_3] -> Divide5/1
  [IH1_3] -> Divide5/2
  [V_Real_Grid_Grid] -> Divide7/1
  [I_Real_Grid_Grid] -> Divide7/2
  Divide7/1 -> [P_Real_Grid]
  Discrete PID Controller5/1 -> MATLAB Function6/1(u)
  MATLAB Function6/1(y) -> PWM Generator (DC-DC)5/1
  Discrete PID Controller3/1 -> MATLAB Function4/1(u)
  MATLAB Function4/1(y) -> PWM Generator (DC-DC)8/1
  PWM Generator (DC-DC)8/1 -> [battery_buck_pwm]
  [V_PV_1] -> MATLAB Function7/1(V_PV_1)
  [V_Wind] -> MATLAB Function7/2(V_Wind)
  MATLAB Function7/1(Wind_Breaker_Boost_Signal_Out) -> PWM Generator (DC-DC)6/1
  [V_PV_1] -> MATLAB Function8/2(V_PV_1)
  MATLAB Function8/1(Wind_Breaker_Boost_Signal_Out) -> PWM Generator (DC-DC)4/1
  Constant3/1 -> MATLAB Function8/1(Sixty)
  PWM Generator (DC-DC)4/1 -> [BH2]
  Permanent Magnet Synchronous Machine/1 -> Gain/1
  [P1_C1] -> Breaker19/1
  [Grid_Energy_Trading_Breaker] -> ?
  MATLAB Function5/1(Fault_Signal) -> [Fault_Signal]
  [V_Fault] -> Divide2/1
  [Fault_Signal] -> ?
  [I_Fault] -> MATLAB Function5/1(I_Fault)
  Divide2/1 -> [Power_Fault]
  [I_Fault] -> Divide2/2
  Three-Phase V-I Measurement5/1 -> [V_Fault]
  Three-Phase V-I Measurement5/2 -> [I_Fault]
  Centralized System/8(H1_B_Ground_Discharge) -> [H1_B_Ground_Discharge]
  Constant4/1 -> Centralized System/2(P_load)
  Centralized System/4(H1_Grid_Breaker) -> [H1_Grid_Breaker]
  Centralized System/1(H1_Pv_Breaker) -> [H1_Pv_Breaker]
  [Battery_Passing_Voltage] -> Centralized System/8(Battery_Passing_Voltage)
  [V_PV_1] -> Centralized System/6(V_PV_1)
  [SOCbH1] -> Centralized System/3(SOCbH1)
  Centralized System/6(Bi_B_Breaker_Discharge_Boost) -> [Bi_B_Breaker_Discharge_Boost]
  [V_Wind] -> Centralized System/7(V_Wind)
  [P_Wind] -> Centralized System/4(P_Wind)
  Centralized System/11(Wind_Breaker_Buck) -> [Wind_Breaker_Buck]
  Centralized System/10(Wind_Breaker_Boost) -> [Wind_Breaker_Boost]
  Centralized System/14(P1_C1) -> [P1_C1]
  Centralized System/2(Bi_B_Charge_Breaker_Buck) -> [Bi_B_Charge_Breaker_Buck]
  Centralized System/13(Wind_Power_Battery_Breaker_Buck) -> [Wind_Power_Battery_Breaker_Buck]
  Centralized System/7(Bi_B_Breaker_Discharge_Buck) -> [Bi_B_Breaker_Discharge_Buck]
  Centralized System/5(H1_Grid_Circuit_Breaker) -> [H1_Grid_Circuit_Breaker]
  [P_Pv] -> Centralized System/1(P_Pv)
  [P_Real_Grid] -> Centralized System/5(P_Real_Grid)
  Centralized System/12(Wind_Power_Battery_Breaker_Boost) -> [Wind_Power_Battery_Breaker_Boost]
  Centralized System/3(Bi_B_Charge_Breaker_Boost) -> [Bi_B_Charge_Breaker_Boost]
  Centralized System/9(Grid_Energy_Trading_Breaker) -> [Grid_Energy_Trading_Breaker]
  connections:
  Three-Phase Breaker/LConn1 -- Three-Phase V-I Measurement/RConn1
  Three-Phase Series RLC Load/LConn3 -- Three phase Inductor removes ripples2/RConn3 -- Three phase Inductor removes ripples3/LConn3
  Three-Phase Breaker/LConn3 -- Three-Phase V-I Measurement/RConn3
  CAPACITOR 3/LConn1 -- Voltage Measurement1/LConn1 -- Current Measurement2/LConn1 -- Diode1/RConn1
  Three-Phase V-I Measurement1/RConn1 -- Three-Phase Breaker3/LConn1 -- Three-Phase Breaker2/LConn1
  Three-Phase Series RLC Load/LConn1 -- Three phase Inductor removes ripples3/LConn1 -- Three phase Inductor removes ripples2/RConn1
  Three-Phase Breaker2/RConn3 -- Three-Phase V-I Measurement2/RConn3 -- Three phase Inductor removes ripples2/LConn3
  Three-Phase Breaker/LConn2 -- Three-Phase V-I Measurement/RConn2
  Three phase Inductor removes ripples1/LConn2 -- Three-Phase V-I Measurement/LConn2 -- Three phase Inductor removes ripples/RConn2
  CAPACITOR 2/RConn1 -- Diode1/LConn1 -- IGBT/Diode/LConn1
  Three phase Inductor removes ripples3/RConn2 -- Three phase Inductor removes ripples3/RConn1 -- Ground1/LConn1 -- Three phase Inductor removes ripples3/RConn3
  Three-Phase Breaker/RConn1 -- Three-Phase V-I Measurement1/LConn1
  Three phase Inductor removes ripples1/LConn1 -- Three-Phase V-I Measurement/LConn1 -- Three phase Inductor removes ripples/RConn1
  Three phase Inductor removes ripples/LConn2 -- Universal Bridge/LConn2
  Three phase Inductor removes ripples/LConn1 -- Universal Bridge/LConn1
  Three-Phase Series RLC Load/LConn2 -- Three phase Inductor removes ripples2/RConn2 -- Three phase Inductor removes ripples3/LConn2
  Three-Phase Breaker2/LConn2 -- Three-Phase Breaker3/LConn2 -- Three-Phase V-I Measurement1/RConn2
  Three-Phase V-I Measurement1/RConn3 -- Three-Phase Breaker3/LConn3 -- Three-Phase Breaker2/LConn3
  Three-Phase Breaker/RConn3 -- Three-Phase V-I Measurement1/LConn3
  Three phase Inductor removes ripples/LConn3 -- Universal Bridge/LConn3
  Ground/LConn1 -- Three phase Inductor removes ripples1/RConn1 -- Three phase Inductor removes ripples1/RConn3 -- Three phase Inductor removes ripples1/RConn2
  Three phase Inductor removes ripples1/LConn3 -- Three-Phase V-I Measurement/LConn3 -- Three phase Inductor removes ripples/RConn3
  CAPACITOR 1/LConn1 -- CAPACITOR 2/LConn1 -- PV Array/RConn1
  Three-Phase Breaker2/RConn1 -- Three-Phase V-I Measurement2/RConn1 -- Three phase Inductor removes ripples2/LConn1
  Three-Phase Breaker2/RConn2 -- Three-Phase V-I Measurement2/RConn2 -- Three phase Inductor removes ripples2/LConn2
  Three-Phase Breaker/RConn2 -- Three-Phase V-I Measurement1/LConn2
  Breaker1/LConn1 -- Current Measurement2/RConn1
  IGBT/Diode1/RConn1 -- CAPACITOR 6/LConn1 -- IGBT/Diode2/LConn1
  CAPACITOR 5/LConn1 -- Battery/LConn1 -- Breaker5/LConn1 -- Breaker4/LConn1 -- CAPACITOR 6/RConn1
  Breaker10/RConn1 -- CAPACITOR 17/LConn1 -- CAPACITOR 18/LConn1
  Thyristor/RConn1 -- CAPACITOR 8/LConn1 -- CAPACITOR 7/LConn1 -- Thyristor4/RConn1 -- Thyristor5/RConn1
  Breaker5/RConn1 -- Mosfet1/LConn1
  Breaker4/RConn1 -- CAPACITOR 11/LConn1 -- CAPACITOR 10/LConn1
  IGBT/Diode4/LConn1 -- Diode3/LConn1 -- CAPACITOR 11/RConn1
  Three-Phase Breaker1/RConn1 -- Three-Phase V-I Measurement2/LConn1
  Three-Phase Breaker1/RConn2 -- Three-Phase V-I Measurement2/LConn2
  Three-Phase Breaker1/RConn3 -- Three-Phase V-I Measurement2/LConn3
  Three-Phase Breaker3/RConn2 -- Three-Phase V-I Measurement3/LConn2
  Three-Phase Breaker3/RConn1 -- Three-Phase V-I Measurement3/LConn1
  Three-Phase Breaker3/RConn3 -- Three-Phase V-I Measurement3/LConn3
  Three-Phase V-I Measurement3/RConn1 -- Three-Phase Source1/RConn1
  Three-Phase V-I Measurement3/RConn2 -- Three-Phase Source1/RConn2
  Three-Phase V-I Measurement3/RConn3 -- Three-Phase Source1/RConn3
  Three-Phase Breaker1/LConn1 -- Three-Phase V-I Measurement4/RConn1
  Three-Phase Breaker1/LConn2 -- Three-Phase V-I Measurement4/RConn2
  Three-Phase Breaker1/LConn3 -- Three-Phase V-I Measurement4/RConn3
  Three-Phase V-I Measurement4/LConn1 -- A/RConn1
  Three-Phase V-I Measurement4/LConn2 -- B/RConn1
  Three-Phase V-I Measurement4/LConn3 -- C/RConn1
  Thyristor/LConn1 -- Thyristor3/RConn1 -- Permanent Magnet Synchronous Machine/LConn1
  Thyristor5/LConn1 -- Thyristor2/RConn1 -- Permanent Magnet Synchronous Machine/LConn2
  Thyristor4/LConn1 -- Permanent Magnet Synchronous Machine/LConn3 -- Thyristor1/RConn1
  Current Measurement1/LConn1 -- Voltage Measurement3/LConn1 -- CAPACITOR 8/RConn1
  Breaker3/LConn1 -- CAPACITOR 5/RConn1 -- IGBT/Diode2/RConn1 -- Voltage Measurement/LConn2 -- CAPACITOR 4/RConn1 -- Voltage Measurement1/LConn2 -- Subsystem/LConn1 -- CAPACITOR 14/RConn1 -- CAPACITOR 9/RConn1 -- Voltage Measurement3/LConn2 -- CAPACITOR 7/RConn1 -- Thyristor1/LConn1 -- Thyristor3/LConn1 -- Thyristor2/LConn1 -- IGBT/Diode3/RConn1 -- Voltage Measurement2/LConn2 -- Universal Bridge/RConn2 -- Voltage Measurement4/LConn2 -- CAPACITOR 16/RConn1 -- CAPACITOR 1/RConn1 -- PV Array/RConn2 -- IGBT/Diode/RConn1 -- CAPACITOR 3/RConn1 -- CAPACITOR 17/RConn1 -- IGBT/Diode5/RConn1 -- CAPACITOR 19/RConn1 -- Battery/LConn2
  Current Measurement3/RConn1 -- Universal Bridge/RConn1
  Mosfet/LConn1 -- Breaker2/RConn1
  Breaker6/LConn1 -- Current Measurement1/RConn1 -- Breaker7/LConn1
  Breaker6/RConn1 -- CAPACITOR 13/LConn1 -- CAPACITOR 9/LConn1
  CAPACITOR 13/RConn1 -- IGBT/Diode3/LConn1 -- Diode2/LConn1
  Mosfet2/LConn1 -- Breaker7/RConn1
  IGBT/Diode4/RConn1 -- CAPACITOR 10/RConn1 -- Breaker3/RConn1 -- CAPACITOR 16/LConn1 -- CAPACITOR 12/RConn1
  Breaker1/RConn1 -- Breaker19/LConn1 -- Current Measurement3/LConn1 -- Voltage Measurement4/LConn1 -- Mosfet2/RConn1 -- Breaker9/LConn1 -- CAPACITOR 14/LConn1 -- Diode2/RConn1 -- Breaker8/LConn1 -- Mosfet1/RConn1 -- Diode3/RConn1 -- CAPACITOR 12/LConn1 -- CAPACITOR 4/LConn1 -- Breaker8/RConn1 -- Voltage Measurement2/LConn1 -- Breaker9/RConn1 -- Breaker2/LConn1 -- Breaker10/LConn1
  Voltage Measurement/LConn1 -- Diode4/RConn1 -- CAPACITOR 19/LConn1 -- Mosfet/RConn1 -- IGBT/Diode1/LConn1
  IGBT/Diode5/LConn1 -- CAPACITOR 18/RConn1 -- Diode4/LConn1
  Breaker19/RConn1 -- Subsystem/LConn2
  Three-Phase Breaker4/RConn2 -- Subsystem/LConn4 -- Three-Phase V-I Measurement5/LConn2
  Three-Phase Breaker4/RConn1 -- Subsystem/LConn3 -- Three-Phase V-I Measurement5/LConn1
  Three-Phase Breaker4/RConn3 -- Subsystem/LConn5 -- Three-Phase V-I Measurement5/LConn3
  Three-Phase V-I Measurement5/RConn1 -- Three-Phase Fault/LConn1
  Three-Phase V-I Measurement5/RConn2 -- Three-Phase Fault/LConn2
  Three-Phase Breaker4/LConn2 -- B1/RConn1
  Three-Phase Breaker4/LConn1 -- A1/RConn1
  Three-Phase Breaker4/LConn3 -- C1/RConn1
  Three-Phase V-I Measurement5/RConn3 -- Three-Phase Fault/LConn3
